simulink model "current_pi_saturation_test_model"  (R2023b)
settings: Solver=FixedStepDiscrete  StartTime=0.0  StopTime=current_pi_sat_test.simcfg.stop_time  FixedStep=current_pi_simcfg.Ts_ctrl  RelTol=1e-3
values from neighbouring files (symbols this model uses):
  Kaw_id = 400.0    [current_pi_interface.sldd]
  Kaw_iq = 400.0    [current_pi_interface.sldd]
  Ki_id = 1072.4140625    [current_pi_interface.sldd]
  Ki_iq = 1072.4140625    [current_pi_interface.sldd]
  Kp_id = 1.3320353031158447    [current_pi_interface.sldd]
  Kp_iq = 1.3320353031158447    [current_pi_interface.sldd]
  VLimitRatio = 0.57700002193450928    [current_pi_interface.sldd]
undefined symbols (not defined in the file or in its folder): current_pi_sat_test, current_pi_simcfg
settings Model: DataDictionary=current_pi_interface.sldd  Creator=user  LastModifiedBy=user
settings OptimizationCC: EnhancedBackFolding=on  PassReuseOutputArgsAs=Individual arguments  ZeroExternalMemoryAtStartup=off  ZeroInternalMemoryAtStartup=off  OptimizeBlockOrder=speed  DifferentSizesBufferReuse=on  OptimizationCustomize=off  EfficientTunableParamExpr=on
settings DebuggingCC: ParameterTunabilityLossMsg=error
settings HardwareCC: ProdBitPerPointer=32  ProdBitPerSizeT=32  ProdBitPerPtrDiffT=32  ProdLargestAtomicInteger=Long  ProdLargestAtomicFloat=Double  ProdWordSize=32  ProdHWDeviceType=ARM Compatible->ARM Cortex  TargetLargestAtomicInteger=Long  TargetLargestAtomicFloat=Double  TargetIntDivRoundTo=Zero  TargetEndianess=LittleEndian  TargetHWDeviceType=ARM Compatible->ARM Cortex  ProdEqTarget=off
settings SFSimCC: MATLABDynamicMemAlloc=off
settings RTWCC: Description=Embedded Coder  SystemTargetFile=ert.tlc  GenCodeOnly=on  TemplateMakefile=ert_default_tmf  RTWVerbose=off
settings CodeAppCC: ForceParamTrailComments=on  IgnoreCustomStorageClasses=off  OperatorAnnotations=on  SimulinkDataObjDesc=on  SFDataObjDesc=on  InsertBlockDesc=on
settings ERTTargetCC: TargetLangStandard=C99 (ISO)  ERTCustomFileTemplate=example_file_process.tlc

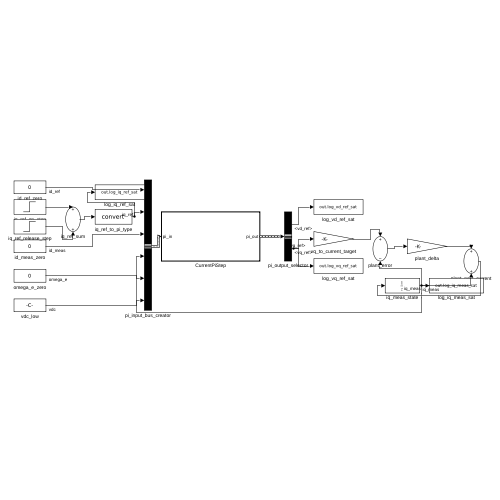
[thumbnail: Simulink's stored preview of the top-level diagram]
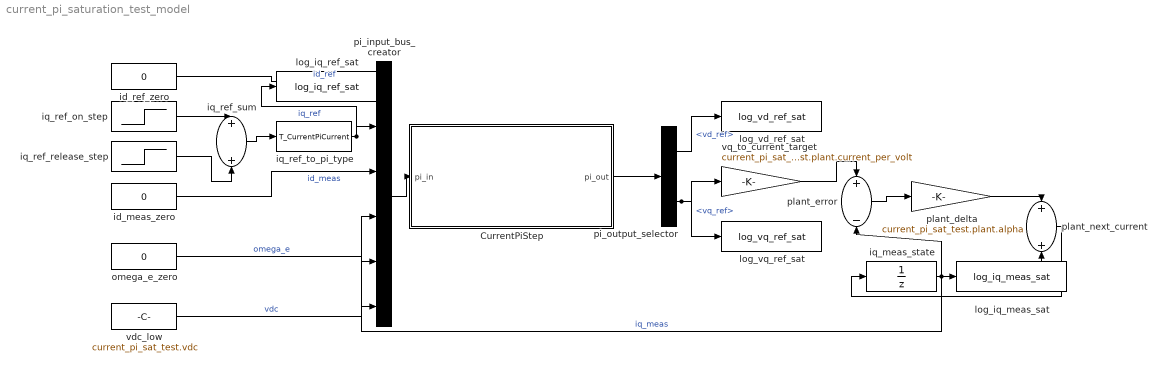
== system current_pi_saturation_test_model ==
  CurrentPiStep : Subsystem  TreatAsAtomicUnit=on  RTWFcnName=CurrentPiStep  RTWFileName=CurrentPiStep
      settings: RTWFcnNameOpts=User specified  RTWFileNameOpts=User specified
  id_meas_zero : Constant  Value=0  OutDataTypeStr=T_CurrentPiCurrent  SampleTime=current_pi_simcfg.Ts_ctrl
  id_ref_zero : Constant  Value=0  OutDataTypeStr=T_CurrentPiCurrent  SampleTime=current_pi_simcfg.Ts_ctrl
  iq_meas_state : UnitDelay  SampleTime=current_pi_simcfg.Ts_ctrl  HasFrameUpgradeWarning=on
  iq_ref_on_step : Step  Time=current_pi_sat_test.ref.on_time  After=current_pi_sat_test.ref.iq_high  SampleTime=current_pi_simcfg.Ts_ctrl
  iq_ref_release_step : Step  Time=current_pi_sat_test.ref.release_time  After=-current_pi_sat_test.ref.iq_high  SampleTime=current_pi_simcfg.Ts_ctrl
  iq_ref_sum : Sum  OutDataTypeStr=T_CurrentPiCurrent  AccumDataTypeStr=T_CurrentPiCurrent
  iq_ref_to_pi_type : DataTypeConversion  OutDataTypeStr=T_CurrentPiCurrent  SaturateOnIntegerOverflow=off  RndMeth=Floor
  log_iq_meas_sat : ToWorkspace  VariableName=log_iq_meas_sat  SaveFormat=Timeseries  SampleTime=-1
  log_iq_ref_sat : ToWorkspace  VariableName=log_iq_ref_sat  SaveFormat=Timeseries  SampleTime=-1
  log_vd_ref_sat : ToWorkspace  VariableName=log_vd_ref_sat  SaveFormat=Timeseries  SampleTime=-1
  log_vq_ref_sat : ToWorkspace  VariableName=log_vq_ref_sat  SaveFormat=Timeseries  SampleTime=-1
  omega_e_zero : Constant  Value=0  OutDataTypeStr=T_CurrentPiSpeed  SampleTime=current_pi_simcfg.Ts_ctrl
  pi_input_bus_creator : BusCreator  Inputs=6  OutDataTypeStr=Bus: current_pi_input_t  NonVirtualBus=on
  pi_output_selector : BusSelector  OutputSignals=vd_ref,vq_ref
  plant_delta : Gain  Gain=current_pi_sat_test.plant.alpha  ParamDataTypeStr=T_CurrentPiGain  OutDataTypeStr=T_CurrentPiCurrent
  plant_error : Sum  Inputs=+-  OutDataTypeStr=T_CurrentPiCurrent  AccumDataTypeStr=T_CurrentPiCurrent
  plant_next_current : Sum  OutDataTypeStr=T_CurrentPiCurrent  AccumDataTypeStr=T_CurrentPiCurrent
  vdc_low : Constant  Value=current_pi_sat_test.vdc  OutDataTypeStr=T_CurrentPiVoltage  SampleTime=current_pi_simcfg.Ts_ctrl
  vq_to_current_target : Gain  Gain=current_pi_sat_test.plant.current_per_volt  ParamDataTypeStr=T_CurrentPiGain  OutDataTypeStr=T_CurrentPiCurrent
  wires:
  CurrentPiStep/1(pi_out) -> pi_output_selector/1
  pi_output_selector/2 -> vq_to_current_target/1, log_vq_ref_sat/1  "<vq_ref>"
  vq_to_current_target/1 -> plant_error/1
  iq_meas_state/1 -> plant_error/2, plant_next_current/2, pi_input_bus_creator/4, log_iq_meas_sat/1  "iq_meas"
  plant_error/1 -> plant_delta/1
  plant_delta/1 -> plant_next_current/1
  plant_next_current/1 -> iq_meas_state/1
  iq_ref_on_step/1 -> iq_ref_sum/1
  iq_ref_release_step/1 -> iq_ref_sum/2
  iq_ref_sum/1 -> iq_ref_to_pi_type/1
  id_ref_zero/1 -> pi_input_bus_creator/1  "id_ref"
  iq_ref_to_pi_type/1 -> pi_input_bus_creator/2, log_iq_ref_sat/1  "iq_ref"
  id_meas_zero/1 -> pi_input_bus_creator/3  "id_meas"
  omega_e_zero/1 -> pi_input_bus_creator/5  "omega_e"
  vdc_low/1 -> pi_input_bus_creator/6  "vdc"
  pi_input_bus_creator/1 -> CurrentPiStep/1(pi_in)
  pi_output_selector/1 -> log_vd_ref_sat/1  "<vd_ref>"

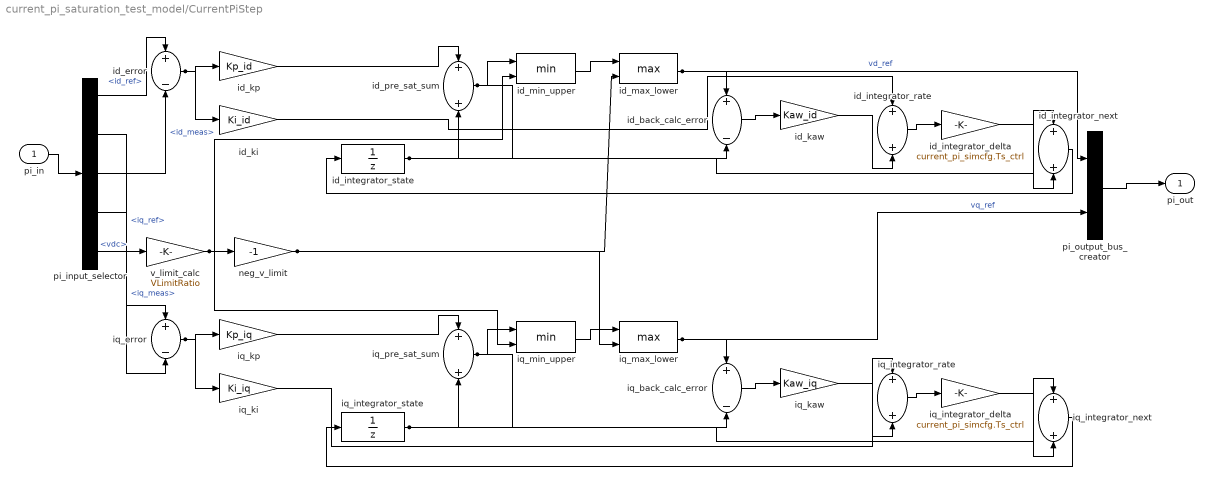
== system current_pi_saturation_test_model/CurrentPiStep ==
  pi_in : Inport  OutDataTypeStr=Bus: current_pi_input_t  BusOutputAsStruct=on
  id_back_calc_error : Sum  Inputs=+-  OutDataTypeStr=T_CurrentPiVoltage  AccumDataTypeStr=T_CurrentPiVoltage
  id_error : Sum  Inputs=+-  OutDataTypeStr=T_CurrentPiCurrent  AccumDataTypeStr=T_CurrentPiCurrent
  id_integrator_delta : Gain  Gain=current_pi_simcfg.Ts_ctrl  ParamDataTypeStr=T_CurrentPiFloat  OutDataTypeStr=T_CurrentPiVoltage
  id_integrator_next : Sum  OutDataTypeStr=T_CurrentPiVoltage  AccumDataTypeStr=T_CurrentPiVoltage
  id_integrator_rate : Sum  OutDataTypeStr=T_CurrentPiVoltage  AccumDataTypeStr=T_CurrentPiVoltage
  id_integrator_state : UnitDelay  SampleTime=current_pi_simcfg.Ts_ctrl  HasFrameUpgradeWarning=on
  id_kaw : Gain  Gain=Kaw_id  ParamDataTypeStr=T_CurrentPiGain  OutDataTypeStr=T_CurrentPiVoltage
  id_ki : Gain  Gain=Ki_id  ParamDataTypeStr=T_CurrentPiGain  OutDataTypeStr=T_CurrentPiVoltage
  id_kp : Gain  Gain=Kp_id  ParamDataTypeStr=T_CurrentPiGain  OutDataTypeStr=T_CurrentPiVoltage
  id_max_lower : MinMax  Function=max  Inputs=2
  id_min_upper : MinMax  Inputs=2
  id_pre_sat_sum : Sum  OutDataTypeStr=T_CurrentPiVoltage  AccumDataTypeStr=T_CurrentPiVoltage
  iq_back_calc_error : Sum  Inputs=+-  OutDataTypeStr=T_CurrentPiVoltage  AccumDataTypeStr=T_CurrentPiVoltage
  iq_error : Sum  Inputs=+-  OutDataTypeStr=T_CurrentPiCurrent  AccumDataTypeStr=T_CurrentPiCurrent
  iq_integrator_delta : Gain  Gain=current_pi_simcfg.Ts_ctrl  ParamDataTypeStr=T_CurrentPiFloat  OutDataTypeStr=T_CurrentPiVoltage
  iq_integrator_next : Sum  OutDataTypeStr=T_CurrentPiVoltage  AccumDataTypeStr=T_CurrentPiVoltage
  iq_integrator_rate : Sum  OutDataTypeStr=T_CurrentPiVoltage  AccumDataTypeStr=T_CurrentPiVoltage
  iq_integrator_state : UnitDelay  SampleTime=current_pi_simcfg.Ts_ctrl  HasFrameUpgradeWarning=on
  iq_kaw : Gain  Gain=Kaw_iq  ParamDataTypeStr=T_CurrentPiGain  OutDataTypeStr=T_CurrentPiVoltage
  iq_ki : Gain  Gain=Ki_iq  ParamDataTypeStr=T_CurrentPiGain  OutDataTypeStr=T_CurrentPiVoltage
  iq_kp : Gain  Gain=Kp_iq  ParamDataTypeStr=T_CurrentPiGain  OutDataTypeStr=T_CurrentPiVoltage
  iq_max_lower : MinMax  Function=max  Inputs=2
  iq_min_upper : MinMax  Inputs=2
  iq_pre_sat_sum : Sum  OutDataTypeStr=T_CurrentPiVoltage  AccumDataTypeStr=T_CurrentPiVoltage
  neg_v_limit : Gain  Gain=-1  ParamDataTypeStr=T_CurrentPiFloat  OutDataTypeStr=T_CurrentPiVoltage
  pi_input_selector : BusSelector  OutputSignals=id_ref,iq_ref,id_meas,iq_meas,vdc
  pi_output_bus_creator : BusCreator  Inputs=2  OutDataTypeStr=Bus: current_pi_output_t  NonVirtualBus=on
  v_limit_calc : Gain  Gain=VLimitRatio  ParamDataTypeStr=T_CurrentPiGain  OutDataTypeStr=T_CurrentPiVoltage
  pi_out : Outport  OutDataTypeStr=Bus: current_pi_output_t
  wires:
  pi_output_bus_creator/1 -> pi_out/1
  iq_integrator_next/1 -> iq_integrator_state/1
  iq_integrator_delta/1 -> iq_integrator_next/2
  iq_integrator_rate/1 -> iq_integrator_delta/1
  iq_kaw/1 -> iq_integrator_rate/2
  iq_ki/1 -> iq_integrator_rate/1
  iq_back_calc_error/1 -> iq_kaw/1
  iq_max_lower/1 -> pi_output_bus_creator/2, iq_back_calc_error/1  "vq_ref"
  iq_min_upper/1 -> iq_max_lower/1
  iq_pre_sat_sum/1 -> iq_back_calc_error/2, iq_min_upper/1
  iq_integrator_state/1 -> iq_integrator_next/1, iq_pre_sat_sum/2
  iq_kp/1 -> iq_pre_sat_sum/1
  iq_error/1 -> iq_ki/1, iq_kp/1
  pi_input_selector/4 -> iq_error/2  "<iq_meas>"
  pi_input_selector/2 -> iq_error/1  "<iq_ref>"
  id_integrator_next/1 -> id_integrator_state/1
  id_integrator_delta/1 -> id_integrator_next/2
  id_integrator_rate/1 -> id_integrator_delta/1
  id_kaw/1 -> id_integrator_rate/2
  id_ki/1 -> id_integrator_rate/1
  id_back_calc_error/1 -> id_kaw/1
  id_max_lower/1 -> pi_output_bus_creator/1, id_back_calc_error/1  "vd_ref"
  neg_v_limit/1 -> iq_max_lower/2, id_max_lower/2
  id_min_upper/1 -> id_max_lower/1
  id_pre_sat_sum/1 -> id_back_calc_error/2, id_min_upper/1
  id_integrator_state/1 -> id_integrator_next/1, id_pre_sat_sum/2
  id_kp/1 -> id_pre_sat_sum/1
  id_error/1 -> id_ki/1, id_kp/1
  pi_input_selector/3 -> id_error/2  "<id_meas>"
  pi_input_selector/1 -> id_error/1  "<id_ref>"
  v_limit_calc/1 -> iq_min_upper/2, id_min_upper/2, neg_v_limit/1
  pi_input_selector/5 -> v_limit_calc/1  "<vdc>"
  pi_in/1 -> pi_input_selector/1
